simulink model "Lab_2_First_and_Second_order"  (R2022b)
settings: Solver=VariableStepAuto  StartTime=0.0  StopTime=10.0  RelTol=1e-3
settings Model: Creator=ahmed  LastModifiedBy=ahmed

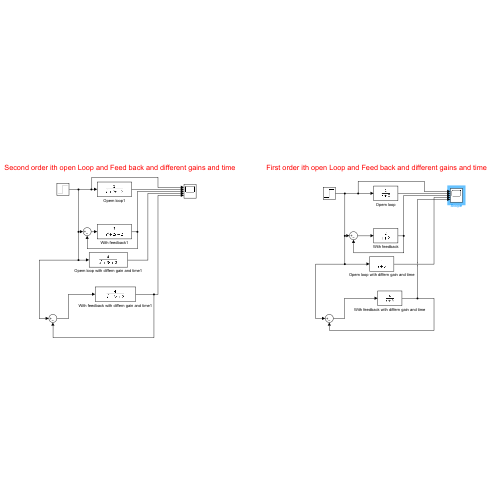
[thumbnail: Simulink's stored preview of the top-level diagram]
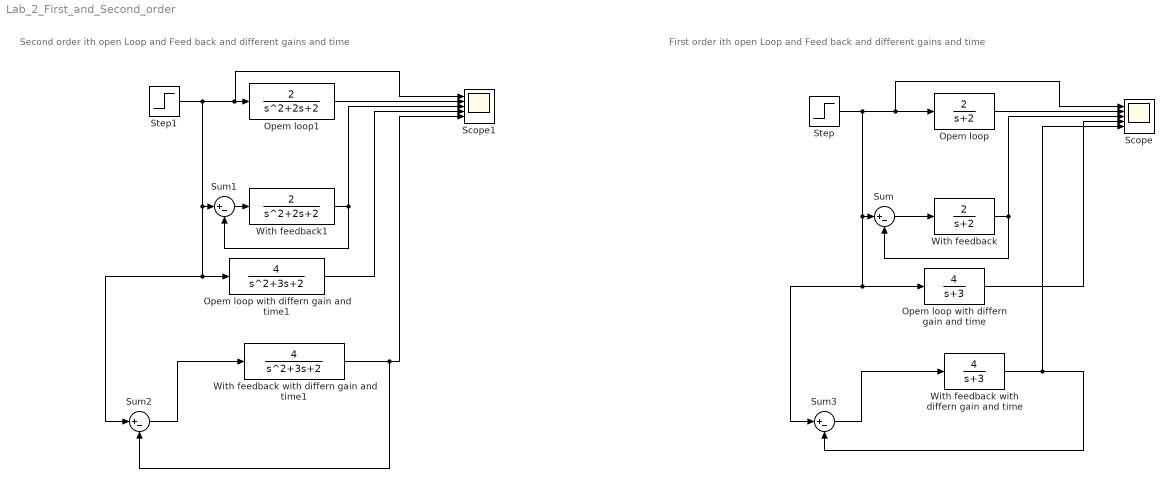
== system Lab_2_First_and_Second_order ==
  note: First order ith open Loop and Feed back and different gains and time
  note: Second order ith open Loop and Feed back and different gains and time
  Opem loop : TransferFcn  Numerator=[2]  Denominator=[1 2]
  Opem loop with differn gain and time : TransferFcn  Numerator=[4]  Denominator=[1 3]
  Opem loop with differn gain and time1 : TransferFcn  Numerator=[4]  Denominator=[1 3 2]
  Opem loop1 : TransferFcn  Numerator=[2]  Denominator=[1 2 2]
  Scope : Scope  NumInputPorts=5
  Scope1 : Scope  NumInputPorts=5
  Step : Step  SampleTime=0
  Step1 : Step  SampleTime=0
  Sum{,1..3} (4 alike) : Sum  Inputs=|+-
  With feedback : TransferFcn  Numerator=[2]  Denominator=[1 2]
  With feedback with differn gain and time : TransferFcn  Numerator=[4]  Denominator=[1 3]
  With feedback with differn gain and time1 : TransferFcn  Numerator=[4]  Denominator=[1 3 2]
  With feedback1 : TransferFcn  Numerator=[2]  Denominator=[1 2 2]
  wires:
  Step/1 -> Opem loop with differn gain and time/1, Sum3/1, Sum/1, Scope/1, Opem loop/1
  Sum/1 -> With feedback/1
  With feedback/1 -> Scope/3, Sum/2
  Opem loop/1 -> Scope/2
  Opem loop with differn gain and time/1 -> Scope/4
  With feedback with differn gain and time/1 -> Sum3/2, Scope/5
  Opem loop1/1 -> Scope1/2
  Step1/1 -> Opem loop with differn gain and time1/1, Sum2/1, Sum1/1, Scope1/1, Opem loop1/1
  With feedback with differn gain and time1/1 -> Sum2/2, Scope1/5
  Sum1/1 -> With feedback1/1
  With feedback1/1 -> Scope1/3, Sum1/2
  Opem loop with differn gain and time1/1 -> Scope1/4
  Sum2/1 -> With feedback with differn gain and time1/1
  Sum3/1 -> With feedback with differn gain and time/1
